simulink model "dpcm075"  (R2019a)
settings: Solver=VariableStepAuto  StartTime=0.0  StopTime=1  RelTol=1e-3
libraries: dspquant2 x2, dsparch4 x1, dspsigops x1
settings Model: Creator=COMMUNCATION LAB  LastModifiedBy=COMMUNCATION LAB

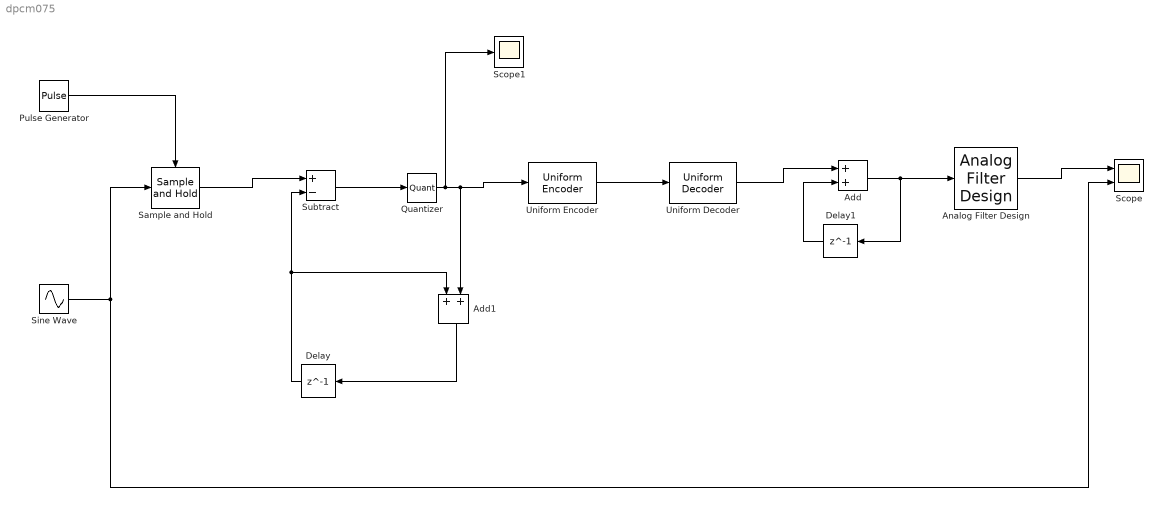
== system dpcm075 ==
  Add : Sum
  Add1 : Sum
  Analog Filter Design : dsparch4/Analog Filter Design  method=Butterworth  filttype=Lowpass  N=16  Wlo=2*pi*40  Whi=80  Rp=2  Rs=40
  Delay : Delay  DelayLength=1  InitialCondition=0
  Delay1 : Delay  DelayLength=1  InitialCondition=0
  Pulse Generator : DiscretePulseGenerator  PulseType=Time based  Amplitude=3  Period=1/750  PulseWidth=5
  Quantizer : Quantizer
  Sample and Hold : dspsigops/Sample and Hold  trig=Rising edge  initCond=0  latchinput=off
  Scope : Scope  NumInputPorts=2
  Scope1 : Scope
  Sine Wave : Sin  Amplitude=3  Frequency=2*pi*20  SampleTime=1/50000
  Subtract : Sum  Inputs=+-
  Uniform Decoder : dspquant2/Uniform Decoder  peak=3  bits=16  overflowMode=Saturate  otype=Double
      settings: SourceProductName=DSP System Toolbox  SourceProductBaseCode=DS
  Uniform Encoder : dspquant2/Uniform Encoder  peak=3  bits=16  otype=Unsigned integer
      settings: SourceProductName=DSP System Toolbox
  wires:
  Pulse Generator/1 -> Sample and Hold/Trigger
  Sine Wave/1 -> Sample and Hold/1, Scope/2
  Sample and Hold/1 -> Subtract/1
  Subtract/1 -> Quantizer/1
  Quantizer/1 -> Scope1/1, Uniform Encoder/1, Add1/2
  Uniform Encoder/1 -> Uniform Decoder/1
  Uniform Decoder/1 -> Add/1
  Add/1 -> Delay1/1, Analog Filter Design/1
  Add1/1 -> Delay/1
  Delay/1 -> Add1/1, Subtract/2
  Delay1/1 -> Add/2
  Analog Filter Design/1 -> Scope/1
